simulink model "Ex9"  (R2020a)
settings: Solver=VariableStepAuto  StartTime=0.0  StopTime=0.2  RelTol=1e-3
libraries: simulink x6, powerlib x5
settings Model: Creator=aishw  LastModifiedBy=aishw

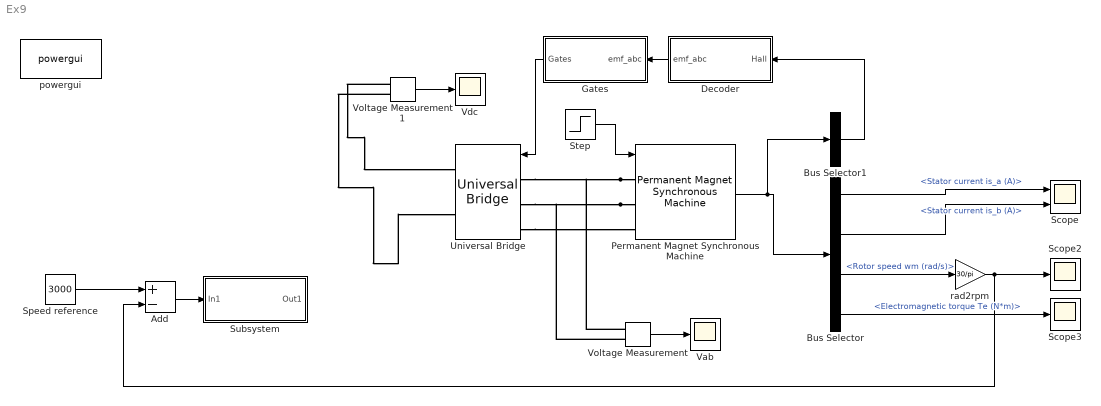
== system Ex9 ==
  Add : Sum  Inputs=+-
  Bus Selector : BusSelector  OutputSignals=Stator current is_a (A),Stator current is_b (A),Rotor speed wm (rad/s),Electromagnetic torque Te (N*m)
  Bus Selector1 : BusSelector  OutputSignals=Hall effect signal h_a,Hall effect signal h_b,Hall effect signal h_c  OutputAsBus=on
  Decoder : Subsystem
  Gates : Subsystem
  Permanent Magnet Synchronous Machine : powerlib/Machines/Permanent Magnet Synchronous Machine  NbPhases=3  FluxDistribution=Trapezoidal  RotorType=Round  MechanicalLoad=Torque Tm  PresetModel=No  ShowDetailedParameters=on  MeasurementBus=off  Resistance=0.0485  Inductance=8.5e-3  dqInductances=[8.5e-3,8.5e-3]  La=0.000395  MachineConstant=Flux linkage established by magnets (V.s)  Flux=0.1194  VoltageCst=100.0283  TorqueCst=0.9552  Flat=120  Mechanical=[0.0027 0.0004924 4 0]  PolePairs=4  InitialConditions=[0,0, 0,0]  InitialConditions5ph=[0 0 0 0 0 0]  RefAngle=90 degrees behind phase A axis (modified Park)  IterativeDiscreteModel=Trapezoidal non iterative  TsBlock=-1  TsPowergui=0
  Scope : Scope  NumInputPorts=2
  Scope2 : Scope
  Scope3 : Scope
  Speed reference : Constant  Value=3000
  Step : Step  Time=0.1  After=3  SampleTime=0
  Subsystem : Subsystem  mask{P=0.013, I=16, sat=[500, -500]}
      mask prompts: P "proportional"; I "Integral"; sat "maximum and minimum"
      mask Display: disp('PI')
  Universal Bridge : powerlib/Power Electronics/Universal Bridge  Arms=3  SnubberResistance=5000  SnubberCapacitance=1e-6  Device=MOSFET / Diodes  Ron=1e-3  Lon=0  ForwardVoltages="[  0  0  ]"  ForwardVoltage=0  GTOparameters=[ 10e-6 , 20e-6 ]  IGBTparameters=[ 1e-6 , 2e-6 ]  Measurements=None  Measurements_2=None  converterType=Rectifier
  Vab : Scope
  Vdc : Scope
  Voltage Measurement : powerlib/Measurements/Voltage Measurement  PhasorSimulation=off  OutputType=Complex  PSBequivalent=0
  Voltage Measurement1 : powerlib/Measurements/Voltage Measurement  PhasorSimulation=off  OutputType=Complex  PSBequivalent=0
  powergui : powerlib/powergui  Priority=1  SimulationMode=Continuous  SampleTime=50e-6  frequency=60  Iterations=50  frequencyindice=0  Pbase=100e6  ErrMax=1e-4  UnitsV=kV  UnitsW=MW  buscounter=0  FunctionMessages=off  echomessages=off  EnableUseOfTLC=off  CurrentSourceSwitches=off  DisableSnubberDevices=off  DisableRonSwitches=off  DisableVfSwitches=off  DisplayEquations=off  AutomaticDiscreteSolvers=off  SolverType=Tustin/Backward Euler (TBE)  Interpol=off  ExternalGateDelay=off  methode=off  Ts=100  x0status=blocks  SPID=on  SwTol=0  HookPort=off  NonlinearTolerance=1e-4  nMaxIteration=100  ContinueOnMaxIteration=off  RestoreLinks=warning  ResistiveCurrentMeasurement=off  Frange=[0:2:500]  Ylog=off  Xlog=on  ShowGrid=off  save=off  variable=ZData  structure=0  ZoomFFT=off  StartTime=0.0  cycles=1  DisplayStyle=1  fundamental=60  FreqAxis=off  MaxFrequency=1000  frequencyindicesteady=1  RmsSteady=1  display=off
  rad2rpm : Gain  Gain=30/pi
  wires:
  Bus Selector1/1 -> Decoder/1(Hall)
  Bus Selector/2 -> Scope/2  "<Stator current is_b (A)>"
  Decoder/1(emf_abc) -> Gates/1(emf_abc)
  Gates/1(Gates) -> Universal Bridge/1
  Permanent Magnet Synchronous Machine/1 -> Bus Selector1/1, Bus Selector/1
  Voltage Measurement1/1 -> Vdc/1
  Bus Selector/3 -> rad2rpm/1  "<Rotor speed wm (rad/s)>"
  Bus Selector/1 -> Scope/1  "<Stator current is_a (A)>"
  Step/1 -> Permanent Magnet Synchronous Machine/1
  Voltage Measurement/1 -> Vab/1
  Bus Selector/4 -> Scope3/1  "<Electromagnetic torque Te (N*m)>"
  Speed reference/1 -> Add/1
  Add/1 -> Subsystem/1(In1)
  rad2rpm/1 -> Add/2, Scope2/1
  connections:
  Voltage Measurement1/LConn2 -- Universal Bridge/RConn2
  Voltage Measurement1/LConn1 -- Universal Bridge/RConn1
  Permanent Magnet Synchronous Machine/LConn1 -- Universal Bridge/LConn1 -- Voltage Measurement/LConn1
  Permanent Magnet Synchronous Machine/LConn2 -- Universal Bridge/LConn2 -- Voltage Measurement/LConn2
  Universal Bridge/LConn3 -- Permanent Magnet Synchronous Machine/LConn3

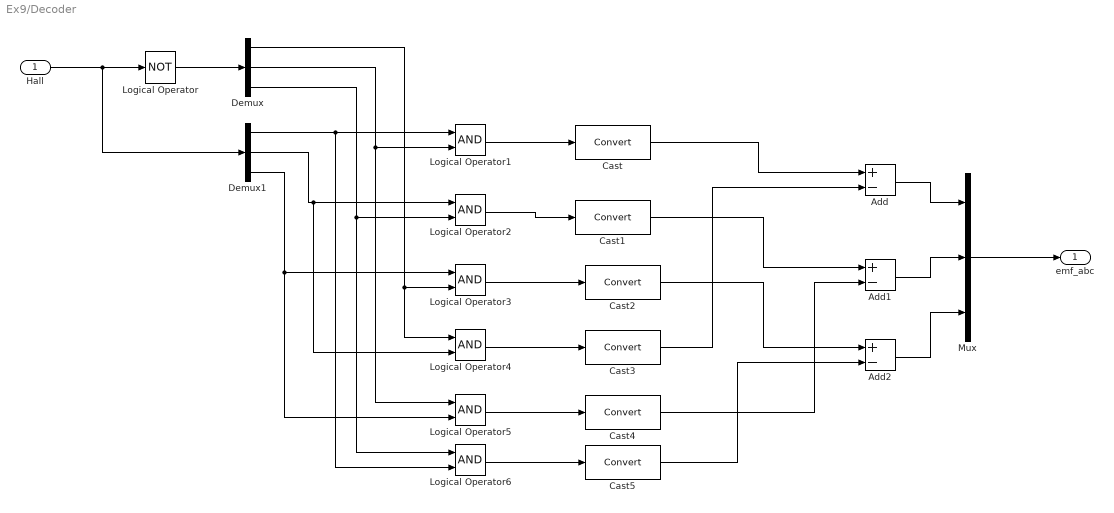
== system Ex9/Decoder ==
  Hall : Inport
  Add : Sum  Inputs=+-
  Add1 : Sum  Inputs=+-
  Add2 : Sum  Inputs=+-
  Cast{,1..5} (6 alike) : DataTypeConversion
  Demux : Demux  Outputs=3
  Demux1 : Demux  Outputs=3
  Logical Operator : Logic  Operator=NOT  AllPortsSameDT=off  OutDataTypeStr=boolean
  Logical Operator{1..6} (6 alike) : Logic  AllPortsSameDT=off  OutDataTypeStr=boolean
  Mux : Mux  Inputs=3
  emf_abc : Outport
  wires:
  Hall/1 -> Demux1/1, Logical Operator/1
  Logical Operator/1 -> Demux/1
  Demux1/1 -> Logical Operator6/2, Logical Operator1/1
  Demux1/2 -> Logical Operator2/1, Logical Operator4/2
  Demux/1 -> Logical Operator3/2, Logical Operator4/1
  Demux/2 -> Logical Operator1/2, Logical Operator5/1
  Demux/3 -> Logical Operator6/1, Logical Operator2/2
  Demux1/3 -> Logical Operator3/1, Logical Operator5/2
  Logical Operator6/1 -> Cast5/1
  Logical Operator5/1 -> Cast4/1
  Logical Operator4/1 -> Cast3/1
  Logical Operator3/1 -> Cast2/1
  Logical Operator2/1 -> Cast1/1
  Logical Operator1/1 -> Cast/1
  Mux/1 -> emf_abc/1
  Add/1 -> Mux/1
  Add1/1 -> Mux/2
  Add2/1 -> Mux/3
  Cast/1 -> Add/1
  Cast1/1 -> Add1/1
  Cast2/1 -> Add2/1
  Cast3/1 -> Add/2
  Cast4/1 -> Add1/2
  Cast5/1 -> Add2/2

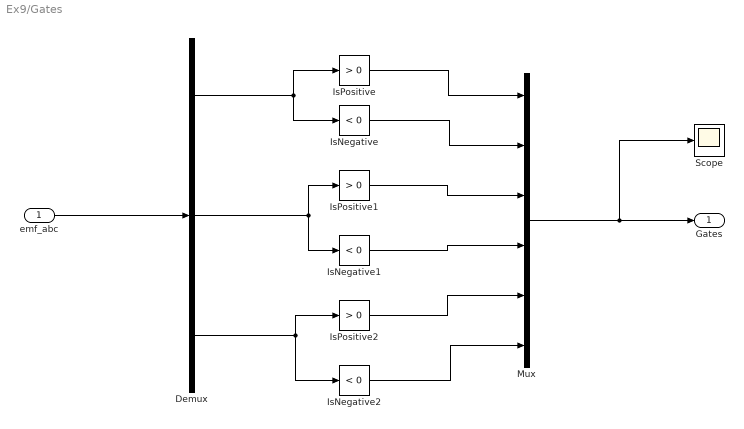
== system Ex9/Gates ==
  emf_abc : Inport
  Demux : Demux  Outputs=3
  IsNegative : simulink/Logic and Bit Operations/Compare To Zero  relop=<  OutDataTypeStr=boolean
  IsNegative1 : simulink/Logic and Bit Operations/Compare To Zero  relop=<  OutDataTypeStr=boolean
  IsNegative2 : simulink/Logic and Bit Operations/Compare To Zero  relop=<  OutDataTypeStr=boolean
  IsPositive : simulink/Logic and Bit Operations/Compare To Zero  relop=>  OutDataTypeStr=boolean
  IsPositive1 : simulink/Logic and Bit Operations/Compare To Zero  relop=>  OutDataTypeStr=boolean
  IsPositive2 : simulink/Logic and Bit Operations/Compare To Zero  relop=>  OutDataTypeStr=boolean
  Mux : Mux  Inputs=6
  Scope : Scope
  Gates : Outport
  wires:
  emf_abc/1 -> Demux/1
  Demux/1 -> IsPositive/1, IsNegative/1
  Demux/2 -> IsNegative1/1, IsPositive1/1
  IsPositive/1 -> Mux/1
  IsNegative/1 -> Mux/2
  IsPositive1/1 -> Mux/3
  IsNegative1/1 -> Mux/4
  IsPositive2/1 -> Mux/5
  IsNegative2/1 -> Mux/6
  Mux/1 -> Scope/1, Gates/1
  Demux/3 -> IsPositive2/1, IsNegative2/1

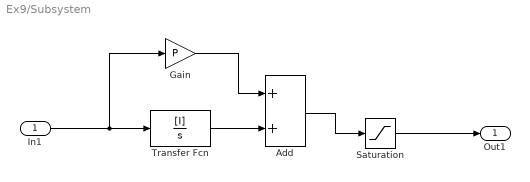
== system Ex9/Subsystem ==
  In1 : Inport
  Add : Sum
  Gain : Gain  Gain=P
  Saturation : Saturate  UpperLimit=500  LowerLimit=-500
  Transfer Fcn : TransferFcn  Numerator=[I]  Denominator=[1 0]
  Out1 : Outport
  wires:
  Add/1 -> Saturation/1
  Saturation/1 -> Out1/1
  Gain/1 -> Add/1
  Transfer Fcn/1 -> Add/2
  In1/1 -> Gain/1, Transfer Fcn/1
